simulink model "untitled_pre"  (R2015a)
settings: Solver=ode45  SolverMode=SingleTasking  StartTime=0.0  StopTime=10.0  RelTol=1e-3
values from neighbouring files (symbols this model uses):
  A = [0 1 0 0 ... (first row only)    [decoupled.m]
  AA = A - B*K    [decoupled.m]
  B = [0 ; -0.286;0;0.386]    [decoupled.m]
  C = [1 0 0 0 ... (first row only)    [decoupled.m]
  D = [0 ; 0 ]    [decoupled.m]
  K = place(A,B,aim_poles)    [decoupled.m]
settings Model: CovMetricSettings=dwe  CovHtmlReporting=off  covSaveCumulativeToWorkspaceVar=off  CovSaveSingleToWorkspaceVar=off  CovExternalEMLEnable=on  Creator=apple  LastModifiedBy=apple
settings DataIOCC: LimitDataPoints=off  SaveFormat=Dataset
settings DebuggingCC: SFUnexpectedBacktrackingDiag=error  SFNoUnconditionalDefaultTransitionDiag=error
settings HardwareCC: ProdBitPerPointer=64  ProdLargestAtomicFloat=Float  ProdIntDivRoundTo=Zero  ProdEndianess=LittleEndian  ProdHWDeviceType=Specified
settings ModelReferenceCC: PropagateSignalLabelsOutOfModel=on
settings GRTTargetCC: TargetLangStandard=C99 (ISO)  GeneratePreprocessorConditionals=Use local settings

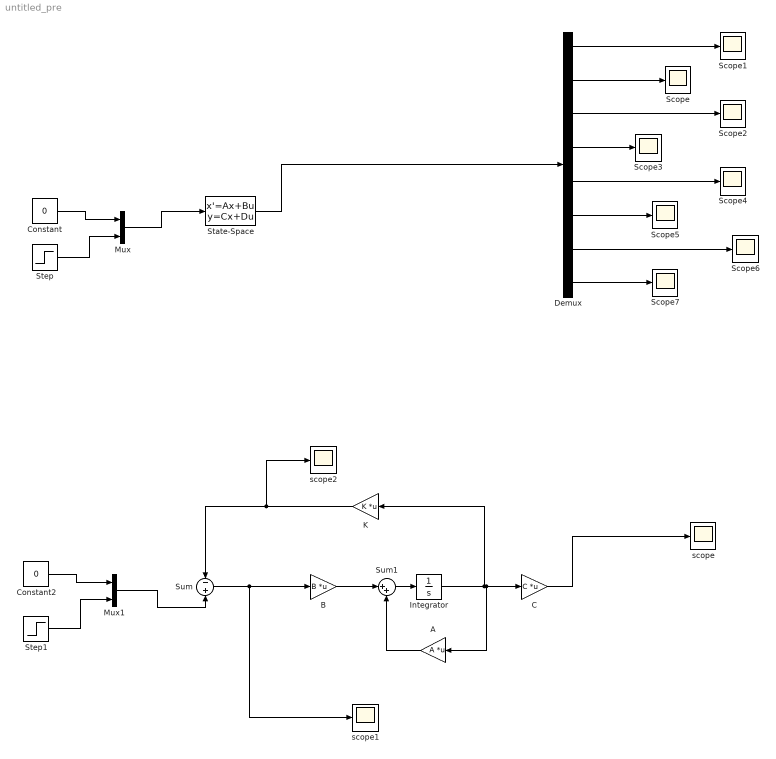
== system untitled_pre ==
  A : Gain  Gain=A  Multiplication=Matrix(K*u)
  B : Gain  Gain=B  Multiplication=Matrix(K*u)
  C : Gain  Gain=C  Multiplication=Matrix(K*u)
  Constant : Constant  Value=0
  Constant2 : Constant  Value=0
  Demux : Demux  Outputs=8
  Integrator : Integrator
  K : Gain  Gain=K  Multiplication=Matrix(K*u)
  Mux : Mux  Inputs=2
  Mux1 : Mux  Inputs=2
  Scope{,1..7} (8 alike) : Scope
      Scope settings: TimeRange=auto  MaxDataPoints=5000  SaveToWorkspace=off  SaveName=ScopeData  YMin=-0.01166  YMax=0.01634  SampleTime=-1
      Scope1 settings: TimeRange=auto  MaxDataPoints=5000  SaveToWorkspace=off  YMin=-0.00029  YMax=0.00044  SampleTime=-1
      Scope2 settings: TimeRange=auto  MaxDataPoints=5000  SaveToWorkspace=off  SaveName=ScopeData2  YMin=-228.94186  YMax=131.75824  SampleTime=-1
      Scope3 settings: TimeRange=auto  MaxDataPoints=5000  SaveToWorkspace=off  SaveName=ScopeData3  YMin=-0.02193  YMax=0.01592  SampleTime=-1
      Scope4 settings: TimeRange=auto  MaxDataPoints=5000  SaveToWorkspace=off  SaveName=ScopeData4  YMin=-0.02931  YMax=0.00326  SampleTime=-1
      Scope5 settings: TimeRange=auto  MaxDataPoints=5000  SaveToWorkspace=off  SaveName=ScopeData5  YMin=-0.32575  YMax=0.04847  SampleTime=-1
      Scope6 settings: TimeRange=auto  MaxDataPoints=5000  SaveToWorkspace=off  SaveName=ScopeData6  YMin=-0.00052  YMax=0.0007  SampleTime=-1
      Scope7 settings: TimeRange=auto  MaxDataPoints=5000  SaveToWorkspace=off  SaveName=ScopeData7  YMin=-0.0194  YMax=0.0264  SampleTime=-1
  State-Space : StateSpace  A=AA  B=B  C=C  D=D  X0=[0 0 1 0 0 0 -1 0]
  Step : Step  After=0  SampleTime=0
  Step1 : Step  Time=0  After=0  SampleTime=0
  Sum : Sum  Inputs=-+
  Sum1 : Sum  Inputs=|++
  scope : Scope
      settings: TimeRange=auto  ShowLegends=on  MaxDataPoints=5000  SaveToWorkspace=off  SaveName=ScopeData10  YMin=-0.32329  YMax=0.06023  SampleTime=-1
  scope1 : Scope
      settings: TimeRange=auto  ShowLegends=on  MaxDataPoints=5000  SaveToWorkspace=off  SaveName=ScopeData8  YMin=-7.41481  YMax=6.1422  SampleTime=-1
  scope2 : Scope
      settings: TimeRange=auto  ShowLegends=on  MaxDataPoints=5000  SaveToWorkspace=off  SaveName=ScopeData9  YMin=-7.41481  YMax=6.1422  SampleTime=-1
  wires:
  State-Space/1 -> Demux/1
  Step/1 -> Mux/2
  Constant/1 -> Mux/1
  Mux/1 -> State-Space/1
  Demux/2 -> Scope/1
  Demux/8 -> Scope7/1
  Demux/1 -> Scope1/1
  Demux/3 -> Scope2/1
  Demux/4 -> Scope3/1
  Demux/5 -> Scope4/1
  Demux/6 -> Scope5/1
  Demux/7 -> Scope6/1
  Sum1/1 -> Integrator/1
  B/1 -> Sum1/1
  A/1 -> Sum1/2
  C/1 -> scope/1
  Integrator/1 -> K/1, A/1, C/1
  Step1/1 -> Mux1/2
  Constant2/1 -> Mux1/1
  Mux1/1 -> Sum/2
  K/1 -> scope2/1, Sum/1
  Sum/1 -> scope1/1, B/1
